simulink subsystem "Circuit_ode_Noise"  (R2022a)
settings: Solver=VariableStepAuto  StartTime=0.0  StopTime=10.0  RelTol=1e-3
values from neighbouring files (symbols this model uses):
  C = [0 0 1]    [DAE_Circuit_main.m]    (also in DAE_Circuit_main_initialStep.m)
  Q = SIM.Q_0*eye(N.inputs)    [DAE_Circuit_main.m]    (also in DAE_Circuit_main_initialStep.m)
  R = SIM.R_0*eye(N.measur)    [DAE_Circuit_main.m]    (also in DAE_Circuit_main_initialStep.m)
undefined symbols (not defined in the file or in its folder): C1, C4, omega, R1, R2, R3, R4, Ts, Vs, x0_2D
settings Model: Creator=tyevans  LastModifiedBy=tyevans

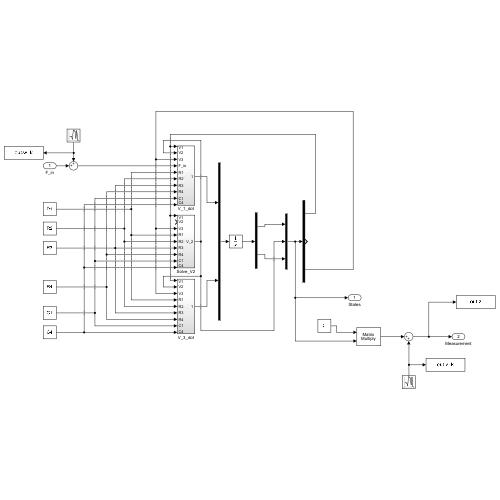
[thumbnail: Simulink's stored preview of the top-level diagram]
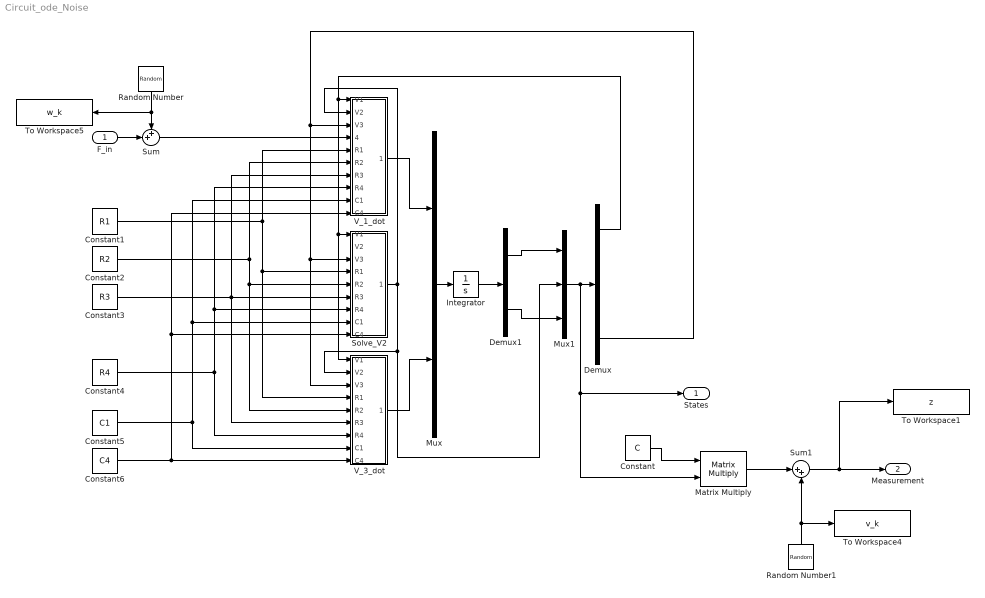
== system Circuit_ode_Noise ==
  F_in : Inport
  Constant : Constant  Value=C  VectorParams1D=off
  Constant1 : Constant  Value=R1  VectorParams1D=off
  Constant2 : Constant  Value=R2  VectorParams1D=off
  Constant3 : Constant  Value=R3  VectorParams1D=off
  Constant4 : Constant  Value=R4  VectorParams1D=off
  Constant5 : Constant  Value=C1  VectorParams1D=off
  Constant6 : Constant  Value=C4  VectorParams1D=off
  Demux : Demux  Outputs=3
  Demux1 : Demux  Outputs=2
  Integrator : Integrator  InitialCondition=x0_2D
  Matrix Multiply : Product  Multiplication=Matrix(*)
  Mux : Mux  Inputs=2
  Mux1 : Mux  Inputs=3
  Random Number : RandomNumber  Variance=Q  SampleTime=Ts  VectorParams1D=off
  Random Number1 : RandomNumber  Variance=diag(R)  SampleTime=Ts
  Solve_V2 : Subsystem
  Sum : Sum  Inputs=++|
  Sum1 : Sum  Inputs=|++
  To Workspace1 : ToWorkspace  VariableName=z  SampleTime=-1
  To Workspace4 : ToWorkspace  VariableName=v_k  SampleTime=-1
  To Workspace5 : ToWorkspace  VariableName=w_k  SampleTime=-1
      settings: Save2DSignal=2-D array (concatenate along first dimension)
  V_1_dot : Subsystem
  V_3_dot : Subsystem
  States : Outport
  Measurement : Outport  Port=2
  wires:
  Demux/1 -> V_1_dot/1(V1), Solve_V2/1(V1), V_3_dot/1(V1)
  V_3_dot/1(Out1) -> Mux/2
  V_1_dot/1(Out1) -> Mux/1
  Demux/3 -> V_1_dot/3(V3), Solve_V2/3(V3), V_3_dot/3(V3)
  Mux/1 -> Integrator/1
  Constant/1 -> Matrix Multiply/1
  Constant6/1 -> Solve_V2/9(C4), V_1_dot/10(C4), V_3_dot/9(C4)
  Constant5/1 -> V_3_dot/8(C1), V_1_dot/9(C1), Solve_V2/8(C1)
  Constant4/1 -> V_1_dot/8(R4), Solve_V2/7(R4), V_3_dot/7(R4)
  Constant3/1 -> Solve_V2/6(R3), V_1_dot/7(R3), V_3_dot/6(R3)
  Constant2/1 -> V_1_dot/6(R2), Solve_V2/5(R2), V_3_dot/5(R2)
  Constant1/1 -> V_1_dot/5(R1), Solve_V2/4(R1), V_3_dot/4(R1)
  Integrator/1 -> Demux1/1
  Demux1/1 -> Mux1/1
  Solve_V2/1(V_2) -> V_1_dot/2(V2), Mux1/2, V_3_dot/2(V2)
  Demux1/2 -> Mux1/3
  Mux1/1 -> Demux/1, States/1, Matrix Multiply/2
  Sum/1 -> V_1_dot/4(F_in)
  F_in/1 -> Sum/2
  Random Number/1 -> To Workspace5/1, Sum/1
  Matrix Multiply/1 -> Sum1/1
  Sum1/1 -> To Workspace1/1, Measurement/1
  Random Number1/1 -> Sum1/2, To Workspace4/1

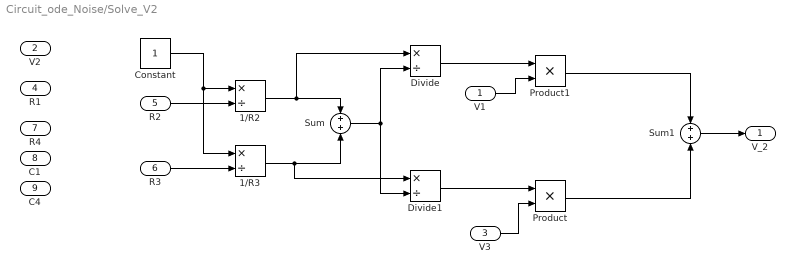
== system Circuit_ode_Noise/Solve_V2 ==
  V1 : Inport
  V2 : Inport  Port=2
  V3 : Inport  Port=3
  R1 : Inport  Port=4
  R2 : Inport  Port=5
  R3 : Inport  Port=6
  R4 : Inport  Port=7
  C1 : Inport  Port=8
  C4 : Inport  Port=9
  1/R2 : Product  Inputs=*/
  1/R3 : Product  Inputs=*/
  Constant : Constant
  Divide : Product  Inputs=*/
  Divide1 : Product  Inputs=*/
  Product : Product
  Product1 : Product
  Sum : Sum
  Sum1 : Sum
  V_2 : Outport
  wires:
  Product1/1 -> Sum1/1
  Product/1 -> Sum1/2
  1/R3/1 -> Divide1/1, Sum/2
  1/R2/1 -> Divide/1, Sum/1
  R3/1 -> 1/R3/2
  R2/1 -> 1/R2/2
  Constant/1 -> 1/R2/1, 1/R3/1
  Sum1/1 -> V_2/1
  Sum/1 -> Divide1/2, Divide/2
  Divide1/1 -> Product/1
  Divide/1 -> Product1/1
  V3/1 -> Product/2
  V1/1 -> Product1/2

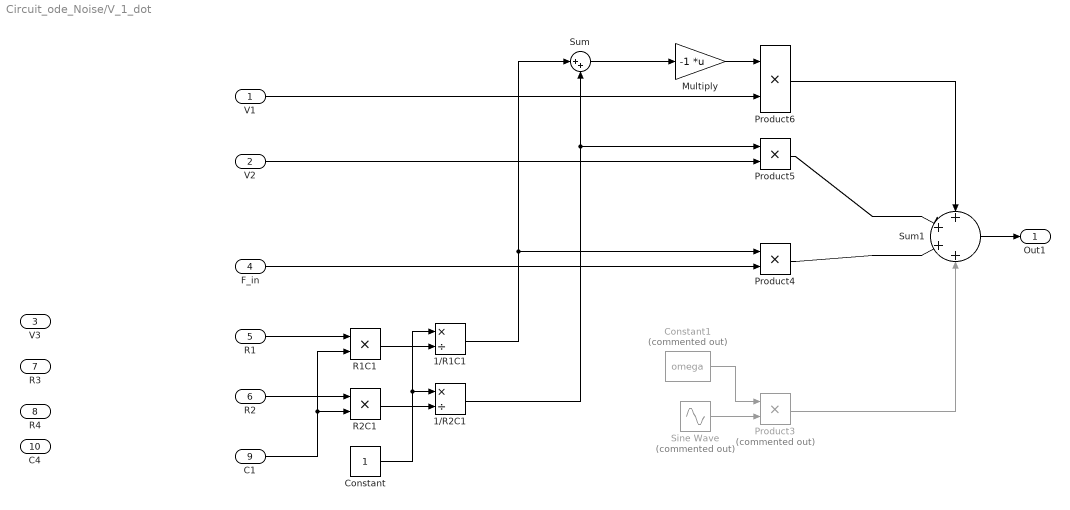
== system Circuit_ode_Noise/V_1_dot ==
  V1 : Inport
  V2 : Inport  Port=2
  V3 : Inport  Port=3
  F_in : Inport  Port=4
  R1 : Inport  Port=5
  R2 : Inport  Port=6
  R3 : Inport  Port=7
  R4 : Inport  Port=8
  C1 : Inport  Port=9
  C4 : Inport  Port=10
  1/R1C1 : Product  Inputs=*/
  1/R2C1 : Product  Inputs=*/
  Constant : Constant
  Constant1 : Constant  Commented=on  Value=omega
  Multiply : Gain  Gain=-1  Multiplication=Matrix(K*u)
  Product3 : Product  Commented=on
  Product4 : Product
  Product5 : Product
  Product6 : Product
  R1C1 : Product
  R2C1 : Product
  Sine Wave : Sin  Commented=on  Amplitude=Vs  Frequency=omega  Phase=pi/2  SampleTime=0  VectorParams1D=off
  Sum : Sum  Inputs=|++
  Sum1 : Sum  Inputs=++++
  Out1 : Outport
  wires:
  Product3/1 -> Sum1/4
  Product4/1 -> Sum1/3
  Product5/1 -> Sum1/2
  Product6/1 -> Sum1/1
  Sum1/1 -> Out1/1
  Constant1/1 -> Product3/1
  Sine Wave/1 -> Product3/2
  F_in/1 -> Product4/2
  V2/1 -> Product5/2
  V1/1 -> Product6/2
  Multiply/1 -> Product6/1
  Sum/1 -> Multiply/1
  1/R2C1/1 -> Sum/2, Product5/1
  1/R1C1/1 -> Sum/1, Product4/1
  R2C1/1 -> 1/R2C1/2
  Constant/1 -> 1/R1C1/1, 1/R2C1/1
  R1C1/1 -> 1/R1C1/2
  R2/1 -> R2C1/1
  C1/1 -> R1C1/2, R2C1/2
  R1/1 -> R1C1/1

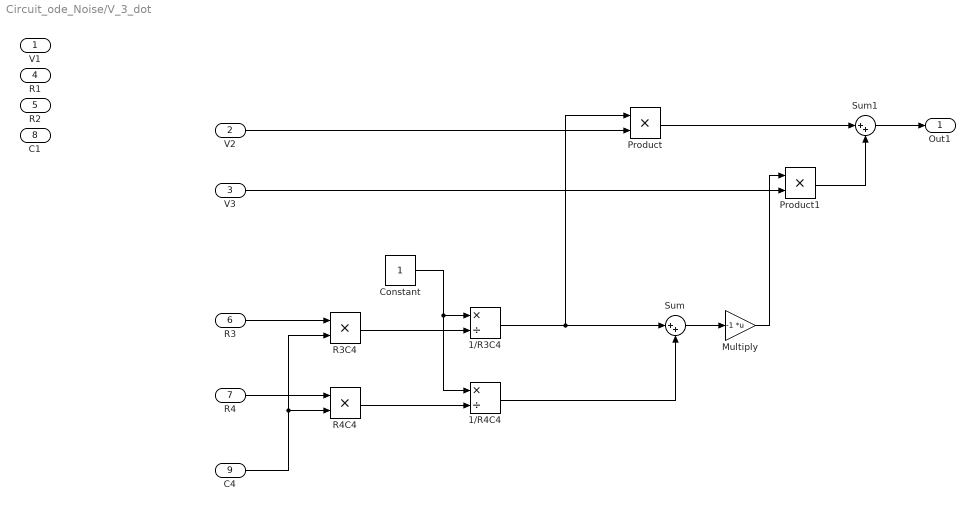
== system Circuit_ode_Noise/V_3_dot ==
  V1 : Inport
  V2 : Inport  Port=2
  V3 : Inport  Port=3
  R1 : Inport  Port=4
  R2 : Inport  Port=5
  R3 : Inport  Port=6
  R4 : Inport  Port=7
  C1 : Inport  Port=8
  C4 : Inport  Port=9
  1/R3C4 : Product  Inputs=*/
  1/R4C4 : Product  Inputs=*/
  Constant : Constant
  Multiply : Gain  Gain=-1  Multiplication=Matrix(K*u)
  Product : Product
  Product1 : Product
  R3C4 : Product
  R4C4 : Product
  Sum : Sum  Inputs=|++
  Sum1 : Sum  Inputs=|++
  Out1 : Outport
  wires:
  Product1/1 -> Sum1/2
  Sum1/1 -> Out1/1
  Product/1 -> Sum1/1
  Multiply/1 -> Product1/1
  V3/1 -> Product1/2
  Sum/1 -> Multiply/1
  1/R4C4/1 -> Sum/2
  1/R3C4/1 -> Product/1, Sum/1
  V2/1 -> Product/2
  R4C4/1 -> 1/R4C4/2
  Constant/1 -> 1/R3C4/1, 1/R4C4/1
  R3C4/1 -> 1/R3C4/2
  R4/1 -> R4C4/1
  C4/1 -> R3C4/2, R4C4/2
  R3/1 -> R3C4/1
